simulink model "mod5counter_simulink"  (R2016a)
settings: Solver=VariableStepAuto  StartTime=0.0  StopTime=100  RelTol=1e-3
model workspace (MAT data in the model file):
  count = Simulink.Parameter
  count.DataType = 'auto'
  count.Dimensions = [0 0]
settings Model: Creator=Admin  LastModifiedBy=Admin
settings DebuggingCC: SignalResolutionControl=TryResolveAll
settings ModelReferenceCC: EnableRefExpFcnMdlSchedulingChecks=off

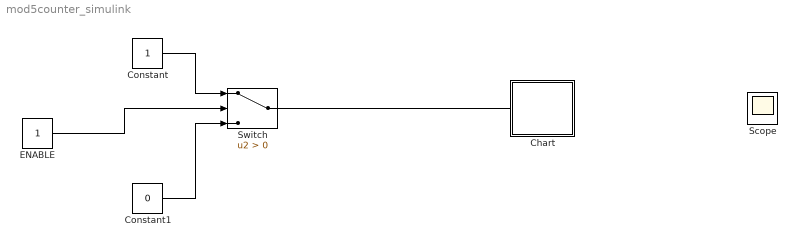
== system mod5counter_simulink ==
  Chart : Stateflow chart  TreatAsAtomicUnit=on
  Constant : Constant
  Constant1 : Constant  Value=0
  ENABLE : Constant
  Scope : Scope
  Switch : Switch  Criteria=u2 > Threshold
  wires:
  Switch/1 -> ?
  Constant/1 -> Switch/1
  Constant1/1 -> Switch/3
  ENABLE/1 -> Switch/2
  ? -> Scope/1

== stateflow chart mod5counter_simulink/Chart ==
